simulink model "satellite3"  (R2025b)
settings: Solver=FixedStepAuto  StartTime=0.0  StopTime=100  FixedStep=dt  MinStep=0.0001  RelTol=1e-3
values from neighbouring files (symbols this model uses):
  A_mw = [ ... (first row only)    [init_params.m]
  A_w = [ ... (first row only)    [init_params.m]
  alpha1 = 0.1    [init_params.m]
  alpha2 = 0.1    [init_params.m]
  angle0 = eAR'    [init_params.m]
  area_d = 4    [init_params.m]
  area_m2 = 0.0127    [init_params.m]
  area_s = 2    [init_params.m]
  ARW_deg_per_sqrt_h = 0.01    [init_params.m]
  B_mw = [ ... (first row only)    [init_params.m]
  bat_bias_on = 0    [init_params.m]
  bat_bias_time = 0    [init_params.m]
  bat_bias_value = 0    [init_params.m]
  bat_cap_on = 0    [init_params.m]
  bat_cap_time = 0    [init_params.m]
  bat_cap_value = 1    [init_params.m]
  beta = 0.3    [init_params.m]
  beta1 = 0.01    [init_params.m]
  beta2 = 0.01    [init_params.m]
  bias0_deg_h = 0.01    [init_params.m]
  C_mw = [ ... (first row only)    [init_params.m]
  Cd = 2.2    [init_params.m]
  Cm = 0.01    [init_params.m]
  cmd_comm = 1    [init_params.m]
  comm_allow = 1    [init_params.m]
  cos_g_max = cos(gamma_max)    [init_params.m]
  Cr = 1.2    [init_params.m]
  cT_deg_on = 0    [init_params.m]
  cT_deg_time = 0    [init_params.m]
  cT_deg_value = 1    [init_params.m]
  cT_delay_on = 0    [init_params.m]
  cT_delay_time = 0    [init_params.m]
  cT_delay_value = 0    [init_params.m]
  cT_drop_on = 0    [init_params.m]
  cT_drop_time = 0    [init_params.m]
  cT_drop_value = 0    [init_params.m]
  cT_lock_on = 0    [init_params.m]
  cT_lock_time = 0    [init_params.m]
  d_c = 2e-5    (= 2e-05)    [init_params.m]
  d_f = 2e-5    (= 2e-05)    [init_params.m]
  D_max = 1    [init_params.m]
  D_thr = 0.4    [init_params.m]
  Delta_D = 0.001    [init_params.m]
  dP_th = 0.05    [init_params.m]
  dss_bias_on = 0    [init_params.m]
  dss_bias_time = 0    [init_params.m]
  dss_bias_value = [0;0;0]    [init_params.m]
  dss_delay_on = 0    [init_params.m]
  dss_delay_time = 0    [init_params.m]
  dss_delay_value = 0    [init_params.m]
  dss_drift_max = 0.1    [init_params.m]
  dss_drift_value = [0;0;0]    [init_params.m]
  dss_drop_on = 0    [init_params.m]
  dss_drop_time = 0    [init_params.m]
  dss_drop_value = [1;0;0]    [init_params.m]
  dss_lock_on = 0    [init_params.m]
  dss_lock_time = 0    [init_params.m]
  dt = 0.1    [init_params.m]
  earth_theta0 = 0    [init_params.m]
  epsilon = 0.01    [init_params.m]
  eT_deg_on = 0    [init_params.m]
  eT_deg_time = 0    [init_params.m]
  eT_deg_value = 1    [init_params.m]
  eT_delay_on = 0    [init_params.m]
  eT_delay_time = 0    [init_params.m]
  eT_delay_value = 0    [init_params.m]
  eT_drop_on = 0    [init_params.m]
  eT_drop_time = 0    [init_params.m]
  eT_drop_value = [0;0;0]    [init_params.m]
  eT_lock_on = 0    [init_params.m]
  eT_lock_time = 0    [init_params.m]
  eta = 0.7    [init_params.m]
  eta_buck = 0.9    [init_params.m]
  eta_et = 0.9    [init_params.m]
  eta_sspa = 0.35    [init_params.m]
  eta_twta = 0.35    [init_params.m]
  f = 2.2e9    (= 2200000000)    [init_params.m]
  f_n_hz = 400    [init_params.m]
  fov = 60*pi/180    (= 1.0471975512)    [init_params.m]
  g0 = 9.80665    [init_params.m]
  G0 = 1366.1    [init_params.m]
  G_sspa_dB = 20    [init_params.m]
  G_twta_dB = 20    [init_params.m]
  Gr_dB = 20    [init_params.m]
  Gt_dB = 3    [init_params.m]
  gyro_bias_on = 0    [init_params.m]
  gyro_bias_time = 0    [init_params.m]
  gyro_bias_value = [0;0;0]    [init_params.m]
  gyro_delay_on = 0    [init_params.m]
  gyro_delay_time = 0    [init_params.m]
  gyro_delay_value = 0    [init_params.m]
  gyro_drift_max = 0.1    [init_params.m]
  gyro_drift_value = [0;0;0]    [init_params.m]
  gyro_drop_on = 0    [init_params.m]
  gyro_drop_time = 0    [init_params.m]
  gyro_drop_value = [0;0;0]    [init_params.m]
  gyro_lock_on = 0    [init_params.m]
  gyro_lock_time = 0    [init_params.m]
  H = 50e3    (= 50000)    [init_params.m]
  h_max = Iw * rpm_max * sqrt(6)    [init_params.m]
  h_ref = 400e3    (= 400000)    [init_params.m]
  I_e = 11    [init_params.m]
  I_gate = 0.5    [init_params.m]
  I_triggle = 8    [init_params.m]
  i_w_max = 2    [init_params.m]
  i_w_min = -2    [init_params.m]
  initial_phase = 0    [init_params.m]
  Isp = 220    [init_params.m]
  Isp_et = 1500    [init_params.m]
  Iw = 0.02    [init_params.m]
  J2 = 1.08262668e-3    (= 0.00108262668)    [init_params.m]
  Jx = 10    [init_params.m]
  Jy = 12    [init_params.m]
  Jz = 8    [init_params.m]
  k_a = 4e-4    (= 0.0004)    [init_params.m]
  k_bias1_deg_h_per_C = 1    [init_params.m]
  k_bias2_deg_h_per_C = 0.0    (= 0)    [init_params.m]
  k_h = -0.05    [init_params.m]
  k_sf1_ppm = 1.0    (= 1)    [init_params.m]
  k_sf2_ppm = 0.0    (= 0)    [init_params.m]
  ... (+207 more)
libraries: matrix_library x25, simulink x14, nesl_utility x4, simulink_extras x3, fl_lib x3, ee_lib x1
(part 2 of 5)

== system satellite3/环境与动力学子系统/行星环境 ==
  x轴坐标 : Inport
  y轴坐标 : Inport  Port=2
  z轴坐标 : Inport  Port=3
  球心距 : Inport  Port=4
  ECI(vx) : Inport  Port=5
  ECI(vy) : Inport  Port=6
  ECI(vz) : Inport  Port=7
  日照标志 : Inport  Port=8
  星日单位向量 : Inport  Port=9
  Add : Sum  Inputs=+++
  Add1 : Sum  Inputs=+++
  Add2 : Sum  Inputs=+++
  J2摄动 : Subsystem
  大气阻力摄动 : Subsystem
  太阳光压摄动 : Subsystem
  ax : Outport
  ay : Outport  Port=2
  az : Outport  Port=3
  wires:
  x轴坐标/1 -> J2摄动/1(x轴坐标), 大气阻力摄动/1(x轴坐标)
  y轴坐标/1 -> J2摄动/2(y轴坐标), 大气阻力摄动/2(y轴坐标)
  z轴坐标/1 -> J2摄动/3(z轴坐标)
  球心距/1 -> 大气阻力摄动/3(球心距), J2摄动/4(球心距)
  ECI(vx)/1 -> 大气阻力摄动/4(vx)
  ECI(vy)/1 -> 大气阻力摄动/5(vy)
  ECI(vz)/1 -> 大气阻力摄动/6(vz)
  J2摄动/1(J2x) -> Add/1
  大气阻力摄动/1(Dx) -> Add/2
  Add/1 -> ax/1
  J2摄动/2(J2y) -> Add1/1
  大气阻力摄动/2(Dy) -> Add1/2
  Add1/1 -> ay/1
  J2摄动/3(J2z) -> Add2/1
  大气阻力摄动/3(Dz) -> Add2/2
  Add2/1 -> az/1
  太阳光压摄动/1(srp_x) -> Add/3
  太阳光压摄动/2(srp_y) -> Add1/3
  太阳光压摄动/3(srp_z) -> Add2/3
  星日单位向量/1 -> 太阳光压摄动/2(hat_r_ss)
  日照标志/1 -> 太阳光压摄动/1(sun_flag)

== system satellite3/电源子系统/充电调节器 ==
  负载电流 : Inport
  太阳能电池电流 : Inport  Port=2
  荷电状态 : Inport  Port=3
  1-SOC2 : Gain  Gain=0.2
  Add : Sum  Inputs=+-
  Add1 : Sum  Inputs=+-
  Constant : Constant  Value=0
  SOC1 : Constant  Value=SOC1
  SOC2 : Constant  Value=SOC2
  SOC_lt_SOC1 : RelationalOperator  Operator=>  OutDataTypeStr=boolean  RndMeth=Simplest  InputSameDT=off
  SOC_lt_SOC2 : RelationalOperator  Operator=>  OutDataTypeStr=boolean  RndMeth=Simplest  InputSameDT=off
  Scope1 : Scope
      settings: ActiveDisplayYMinimum=-0.1607142857142857  ActiveDisplayYMaximum=1.4464285714285716  DataLoggingVariableName=ScopeData43
  Switch : Switch  Criteria=u2 > Threshold  SaturateOnIntegerOverflow=off  InputSameDT=off
  Switch2 : Switch  Threshold=0.2  SaturateOnIntegerOverflow=off  InputSameDT=off
  涓流|稳流 : Switch  Criteria=u2 > Threshold  SaturateOnIntegerOverflow=off  InputSameDT=off
  涓流充电电流 : Constant  Value=0.3
  稳压充电电流 : Product
  稳流|稳压 : Switch  Criteria=u2 > Threshold  SaturateOnIntegerOverflow=off  InputSameDT=off
  稳流充电电流 : Constant  Value=0.6
  净充电电流 : Outport
  wires:
  [one] -> Add1/1
  SOC_lt_SOC2/1 -> 稳流|稳压/2
  1-SOC2/1 -> 稳流|稳压/3
  稳流充电电流/1 -> 稳流|稳压/1
  SOC_lt_SOC1/1 -> 涓流|稳流/2
  Add1/1 -> 1-SOC2/1
  SOC1/1 -> SOC_lt_SOC1/1
  SOC2/1 -> SOC_lt_SOC2/1
  涓流充电电流/1 -> 涓流|稳流/1
  稳流|稳压/1 -> 涓流|稳流/3
  涓流|稳流/1 -> 稳压充电电流/1
  Switch2/1 -> Scope1/1, Switch/3
  荷电状态/1 -> SOC_lt_SOC2/2, SOC_lt_SOC1/2, Switch2/2, Add1/2
  Constant/1 -> Switch2/3
  Add/1 -> Switch/2, 稳压充电电流/2, Switch2/1
  太阳能电池电流/1 -> Add/1
  负载电流/1 -> Add/2
  稳压充电电流/1 -> Switch/1
  Switch/1 -> 净充电电流/1

== system satellite3/电源子系统/太阳能板 ==
  note: V_bus 一旦跌到很低，I_load 变成极大，直接把系统拉飞
  note: 占比法计算负载电阻
      | $I_{load}=\frac{P_{cpl}}{V_{bus}}+\frac{V_{bus}}{R_{load}} \\ R_{load}=\frac{V_{bus,ref}^2}{P_R}=\frac{V_{bus,ref}^2}{\beta P_{load,max}}$
  note: 恒功率负载的“负阻抗”不稳定，当母线电压下降时，负载电流会增大，进一步拉低电压，容易引起母线电压振荡，因此添加电阻性负载
  note: 最简单的光生电流，后续可改为
      | $I_{pannel}=I_{ph}-I_0\left( e^{\frac{V_{pannel}+IR_s}{nV_t}} -1\right)-\frac{V_{pannel}+IR_s}{R_{sh}}$
  日照标志 : Inport
  q : Inport  Port=2
  星日单位矢量 : Inport  Port=3
  V_batt : Inport  Port=4
  电流差 : Inport  Port=5
  P_load : Inport  Port=6
  Gain2 : Gain  Gain=beta
  Gain3 : Gain  Gain=1/R_load
  Product3 : Product  Inputs=*/
  Relay : Relay  OnSwitchValue=V_uvlo_on  OffSwitchValue=V_uvlo_off
  Scope1 : Scope
      settings: ActiveDisplayYMinimum=26.370093999451154  ActiveDisplayYMaximum=30.950942722590582  DataLoggingVariableName=ScopeData29
  Scope3 : Scope
      settings: ActiveDisplayYMinimum=14  ActiveDisplayYMaximum=34  DataLoggingVariableName=ScopeData43
  Scope4 : Scope  NumInputPorts=3
      settings: ActiveDisplayYMinimum=-2.5150334771348364  ActiveDisplayYMaximum=7.0208781354201077  DataLoggingVariableName=ScopeData47
  Sum1 : Sum  Inputs=|++
  太阳板 : Subsystem
  数学保护 : Saturate  UpperLimit=50  LowerLimit=V_bus0
  母线故障 : Subsystem
  蓄电池充电电流 : Outport
  负载电流 : Outport  Port=2
  非欠压 : Outport  Port=3
  wires:
  太阳板/1(太阳板输出电流) -> 蓄电池充电电流/1, Scope4/1
  Sum1/1 -> Scope4/3, 负载电流/1  "I_load"
  q/1 -> 太阳板/1(q)
  日照标志/1 -> 太阳板/2(日照标志)
  母线故障/1(故障值) -> Scope1/1, Relay/1, 太阳板/4(母线电压), 数学保护/1, Gain3/1  "V_bus"
  星日单位矢量/1 -> 太阳板/3(星日单位矢量)
  Gain2/1 -> Product3/1
  Product3/1 -> Sum1/1
  Gain3/1 -> Sum1/2
  数学保护/1 -> Product3/2
  Relay/1 -> 非欠压/1
  P_load/1 -> Gain2/1
  电流差/1 -> Scope4/2
  V_batt/1 -> 母线故障/1(原值)

== system satellite3/电源子系统/姿态确认与控制功耗 ==
  SOC : Inport
  adcs_load : Inport  Port=2
  not_shed : Inport  Port=3
  0.01 : Constant  Commented=on  Value=0.01
  1 : Constant
  AND1 : Logic  Inputs=5  AllPortsSameDT=off  OutDataTypeStr=boolean
  AND2 : Logic  AllPortsSameDT=off  OutDataTypeStr=boolean
  Add2 : Sum
  SOC_adcs_1/0 : Relay  OnSwitchValue=SOC_low_adcs + 0.02  OffSwitchValue=SOC_low_adcs  OutDataTypeStr=boolean
  Switch : Switch  Criteria=u2 > Threshold  Threshold=0.5  SaturateOnIntegerOverflow=off  InputSameDT=off
  T_gt_001 : RelationalOperator  Commented=on  Operator=<=  OutDataTypeStr=boolean  RndMeth=Simplest  InputSameDT=off
  姿态开时负载功耗 : Constant  Value=P_adcs
  adcs_on : Outport
  P_adcs : Outport  Port=2
  wires:
  Switch/1 -> P_adcs/1
  adcs_load/1 -> Add2/1, T_gt_001/2
  AND2/1 -> Switch/2, adcs_on/1
  Add2/1 -> Switch/1
  0.01/1 -> T_gt_001/1
  姿态开时负载功耗/1 -> Add2/2
  [zero] -> Switch/3
  SOC/1 -> SOC_adcs_1/0/1
  SOC_adcs_1/0/1 -> AND2/2
  1/1 -> AND2/1

== system satellite3/电源子系统/推进子系统功耗 ==
  SOC : Inport
  prop_load : Inport  Port=2
  not_shed : Inport  Port=3
  2 : Constant
  AND : Logic  AllPortsSameDT=off  OutDataTypeStr=boolean
  SOC_prop_1/0 : Relay  OnSwitchValue=SOC_low_prop + 0.02  OffSwitchValue=SOC_low_prop  OutDataTypeStr=boolean
  Switch : Switch  Criteria=u2 > Threshold  Threshold=0.5  SaturateOnIntegerOverflow=off  InputSameDT=off
  P_prop : Outport
  prop_on : Outport  Port=2
  wires:
  SOC/1 -> SOC_prop_1/0/1
  AND/1 -> prop_on/1, Switch/2
  Switch/1 -> P_prop/1
  prop_load/1 -> Switch/1
  [zero] -> Switch/3
  SOC_prop_1/0/1 -> AND/1
  2/1 -> AND/2

== system satellite3/电源子系统/蓄电池组 ==
  净充电电流 : Inport
  Add3 : Sum
  Ah2As : Gain  Gain=1/3600
  Constant : Constant  Value=Qbat
  D : Gain  Gain=Rb
  Fcn : Fcn  Expr=24+9*u
  Fcn1 : Fcn  Expr=-7.5*u^3+15*u^2+3.5*u+24
  I_delay : Memory  LinearizeAsDelay=on
  Product : Product  Inputs=*/
  Scope1 : Scope
      settings: ActiveDisplayYMinimum=29.158033567408072  ActiveDisplayYMaximum=29.963419336128545  DataLoggingVariableName=ScopeData27
  Scope2 : Scope
      settings: ActiveDisplayYMinimum=0.59993300420194839  ActiveDisplayYMaximum=0.60060296218246534  DataLoggingVariableName=ScopeData9
  Scope3 : Scope
      settings: ActiveDisplayYMinimum=-2.9294047342041475E-5  ActiveDisplayYMaximum=4.7292744475508951E-5  DataLoggingVariableName=ScopeData51
  int_Q : Integrator  InitialCondition=SOC0*Qbat  LimitOutput=on  UpperSaturationLimit=Qbat  LowerSaturationLimit=0
  蓄电池组故障 : Subsystem
  V_batt : Outport
  电流差 : Outport  Port=2
  SOC : Outport  Port=3
  wires:
  Add3/1 -> V_batt/1
  净充电电流/1 -> I_delay/1
  Fcn1/1 -> Scope1/1, Add3/2
  Product/1 -> Fcn1/1, Scope2/1, SOC/1
  D/1 -> Add3/1
  I_delay/1 -> 电流差/1, Ah2As/1, D/1
  int_Q/1 -> Product/1, Scope3/1
  Ah2As/1 -> int_Q/1
  Constant/1 -> 蓄电池组故障/1(原值)
  蓄电池组故障/1(故障值) -> Product/2

== system satellite3/电源子系统/通信子系统功耗 ==
  note: 因为阴影期 电源更紧张 ：太阳板发电为 0，所有功耗都由电池承担。通信通常是大功耗载荷之一（例如几十瓦到上百瓦），如果阴影期仍高占空比通信，SOC 会更快下滑，导致系统触发保护（关载荷/进 Safe Mode）
  SOC : Inport
  Vizlit : Inport  Port=2
  sunlit : Inport  Port=3
  not_shed : Inport  Port=4
  cmd_comm_on : Inport  Port=5
  1 : Constant
  3 : Constant
  4 : Constant
  AND1 : Logic  Inputs=5  AllPortsSameDT=off  OutDataTypeStr=boolean
  SOC_comm_1/0 : Relay  OnSwitchValue=SOC_low_comm + 0.02  OffSwitchValue=SOC_low_comm
  Switch : Switch  Criteria=u2 > Threshold  Threshold=0.5  SaturateOnIntegerOverflow=off  InputSameDT=off
  通信开时负载功耗 : Constant  Value=P_comm
  comm_on : Outport
  通信功耗 : Outport  Port=2
  wires:
  AND1/1 -> Switch/2, comm_on/1
  sunlit/1 -> AND1/3
  通信开时负载功耗/1 -> Switch/1
  SOC_comm_1/0/1 -> AND1/1
  Switch/1 -> 通信功耗/1
  SOC/1 -> SOC_comm_1/0/1
  Vizlit/1 -> AND1/2
  [zero] -> Switch/3
  cmd_comm_on/1 -> AND1/5
  1/1 -> AND1/4

== system satellite3/通信子系统/SSPA ==
  tx_on : Inport
  Gain : Gain  Gain=0.1
  Gain1 : Gain  Gain=1/eta_sspa
  Math Function : Math  Operator=10^u
  Saturation : Saturate  UpperLimit=P_sspa_dBW  LowerLimit=0
  Sum : Sum  Inputs=|++
  Switch : Switch  Criteria=u2 > Threshold  SaturateOnIntegerOverflow=off  InputSameDT=off
  dbW : Constant  Value=-100
  前级驱动功率 : Constant  Value=P_in_driver_dBW
  小信号增益 : Constant  Value=G_sspa_dB
  Pt_dBW : Outport
  load : Outport  Port=2
  wires:
  前级驱动功率/1 -> Sum/1
  小信号增益/1 -> Sum/2
  Sum/1 -> Saturation/1
  Saturation/1 -> Switch/1
  tx_on/1 -> Switch/2
  dbW/1 -> Switch/3
  Math Function/1 -> Gain1/1
  Gain/1 -> Math Function/1
  Switch/1 -> Gain/1, Pt_dBW/1
  Gain1/1 -> load/1

== system satellite3/通信子系统/TWTA ==
  note: TWTA 往往不是瞬时可用。比如：
      | 发射指令来了后开始计时
      | 计时大于 5 s 才允许输出功率
      | 这会比 SSPA 更贴近工程。
  tx_on : Inport
  Delay1 : Delay  DelayLength=5/dt
  Gain : Gain  Gain=0.1
  Gain1 : Gain  Gain=1/eta_twta
  Math Function : Math  Operator=10^u
  Saturation : Saturate  UpperLimit=P_twta_dBW  LowerLimit=0
  Sum : Sum  Inputs=|++
  Switch : Switch  Criteria=u2 > Threshold  SaturateOnIntegerOverflow=off  InputSameDT=off
  dbW : Constant  Value=-100
  前级驱动功率 : Constant  Value=P_in_driver_dBW
  小信号增益 : Constant  Value=G_twta_dB
  Pt_dBW : Outport
  load : Outport  Port=2
  wires:
  dbW/1 -> Switch/3
  Saturation/1 -> Switch/1
  Sum/1 -> Saturation/1
  小信号增益/1 -> Sum/2
  前级驱动功率/1 -> Sum/1
  Gain1/1 -> load/1
  Math Function/1 -> Gain1/1
  Gain/1 -> Math Function/1
  Delay1/1 -> Pt_dBW/1, Gain/1
  tx_on/1 -> Switch/2
  Switch/1 -> Delay1/1

== system satellite3/通信子系统/向量模长-r ==
  u1 : Inport
  u2 : Inport  Port=2
  u3 : Inport  Port=3
  Add : Sum  Inputs=+++
  Sqrt : Sqrt
  Square : Math  Operator=square
  Square1 : Math  Operator=square
  Square2 : Math  Operator=square
  |u| : Outport
  wires:
  u1/1 -> Square/1
  u2/1 -> Square1/1
  u3/1 -> Square2/1
  Square/1 -> Add/1
  Square1/1 -> Add/2
  Square2/1 -> Add/3
  Add/1 -> Sqrt/1
  Sqrt/1 -> |u|/1

== system satellite3/姿态确定与控制系统/三轴PD控制器/共轭 ==
  u : Inport
  -q1 : Gain  Gain=-1
  -q2 : Gain  Gain=-1
  -q3 : Gain  Gain=-1
  Demux : Demux
  Mux : Mux
  u^-1 : Outport
  wires:
  Mux/1 -> u^-1/1
  Demux/1 -> Mux/1
  Demux/2 -> -q1/1
  -q1/1 -> Mux/2
  Demux/3 -> -q2/1
  -q2/1 -> Mux/3
  Demux/4 -> -q3/1
  -q3/1 -> Mux/4
  u/1 -> Demux/1

== system satellite3/姿态确定与控制系统/三轴PD控制器/四元数乘法 ==
  Q1 : Inport
  Q2 : Inport  Port=2
  Add : Sum  Inputs=3
  Cross Product : matrix_library/Cross Product
  Demux : Demux
  Demux1 : Demux
  Dot Product : DotProduct  OutDataTypeStr=Inherit: Inherit via internal rule
  Mux : Mux  Inputs=2
  Mux1 : Mux  Inputs=3
  Mux2 : Mux  Inputs=3
  Product : Product
  Product1 : Product
  Product2 : Product
  Sum : Sum  Inputs=|+-
  四元数旋转偏差 : Outport
  wires:
  Q1/1 -> Demux/1
  Q2/1 -> Demux1/1
  Mux/1 -> 四元数旋转偏差/1
  Product/1 -> Sum/1
  Demux/1 -> Product1/1, Product/1
  Mux1/1 -> Dot Product/1, Cross Product/1, Product2/2
  Demux1/1 -> Product2/1, Product/2
  Mux2/1 -> Cross Product/2, Dot Product/2, Product1/2
  Sum/1 -> Mux/1
  Dot Product/1 -> Sum/2
  Product2/1 -> Add/2
  Product1/1 -> Add/1
  Cross Product/1 -> Add/3
  Add/1 -> Mux/2
  Demux/2 -> Mux1/1
  Demux/3 -> Mux1/2
  Demux/4 -> Mux1/3
  Demux1/2 -> Mux2/1
  Demux1/3 -> Mux2/2
  Demux1/4 -> Mux2/3

== system satellite3/姿态确定与控制系统/三轴PD控制器/四元数归一化 ==
  In1 : Inport
  Demux1 : Demux
  Mux1 : Mux
  Product{2..5} (4 alike) : Product  Inputs=*/
  向量模长-q : Subsystem
  Out1 : Outport
  wires:
  Demux1/4 -> Product5/1, 向量模长-q/4(u3)
  Product5/1 -> Mux1/4  "q3"
  Demux1/2 -> 向量模长-q/2(u1), Product3/1
  向量模长-q/1(|u|) -> Product3/2, Product4/2, Product5/2, Product2/2
  Demux1/1 -> 向量模长-q/1(u0), Product2/1
  Demux1/3 -> 向量模长-q/3(u2), Product4/1
  Product3/1 -> Mux1/2  "q1"
  Product2/1 -> Mux1/1  "q0"
  Product4/1 -> Mux1/3  "q2"
  Mux1/1 -> Out1/1
  In1/1 -> Demux1/1

== system satellite3/姿态确定与控制系统/三轴姿态动力学子系统/rlg_p ==
  p : Inport
  Lamb激光动力学 : Subsystem
  Sum : Sum  Inputs=+-|
  Terminator : Terminator
  几何参数 : Subsystem
  噪声模型 : Subsystem
  控模与扫模逻辑 : Subsystem
  机械抖动 : Subsystem  Commented=on
  热模型 : Subsystem
  环境温度 : Sin  Amplitude=10  Bias=25  Frequency=(2*pi)/3600  SampleTime=0
  hat_p : Outport
  wires:
  控模与扫模逻辑/1(扫模电压) -> Lamb激光动力学/5(扫模电压)
  Lamb激光动力学/1(相位差变化率) -> 噪声模型/2(相位差变化率)
  热模型/2(温度标度因数) -> Lamb激光动力学/2(温度标度因数)
  噪声模型/1(测量角速度) -> Sum/2, hat_p/1  "测量角速度"
  几何参数/1(标度因数) -> 噪声模型/1(标度因数), 热模型/2(几何标度因数)
  p/1 -> Lamb激光动力学/1(本体角速度), Sum/1  "本体角速度"
  机械抖动/1(抖动角速度) -> Lamb激光动力学/4(抖动角速度)
  热模型/3(温度零偏) -> Lamb激光动力学/3(零偏速率)
  环境温度/1 -> 热模型/1(环境温度-°C)
  Lamb激光动力学/2(光强) -> 控模与扫模逻辑/1(光强)
  Sum/1 -> Terminator/1

== system satellite3/姿态确定与控制系统/三轴姿态动力学子系统/rlg_q ==
  q : Inport
  Lamb激光动力学 : Subsystem
  Sum : Sum  Inputs=+-|
  Terminator : Terminator
  几何参数 : Subsystem
  噪声模型 : Subsystem
  控模与扫模逻辑 : Subsystem
  机械抖动 : Subsystem  Commented=on
  热模型 : Subsystem
  环境温度 : Sin  Amplitude=10  Bias=25  Frequency=(2*pi)/3600  SampleTime=0
  hat_q : Outport
  wires:
  Sum/1 -> Terminator/1
  Lamb激光动力学/2(光强) -> 控模与扫模逻辑/1(光强)
  环境温度/1 -> 热模型/1(环境温度-°C)
  热模型/3(温度零偏) -> Lamb激光动力学/3(零偏速率)
  机械抖动/1(抖动角速度) -> Lamb激光动力学/4(抖动角速度)
  q/1 -> Sum/1, Lamb激光动力学/1(本体角速度)  "本体角速度"
  几何参数/1(标度因数) -> 热模型/2(几何标度因数), 噪声模型/1(标度因数)
  噪声模型/1(测量角速度) -> hat_q/1, Sum/2  "测量角速度"
  热模型/2(温度标度因数) -> Lamb激光动力学/2(温度标度因数)
  Lamb激光动力学/1(相位差变化率) -> 噪声模型/2(相位差变化率)
  控模与扫模逻辑/1(扫模电压) -> Lamb激光动力学/5(扫模电压)

== system satellite3/姿态确定与控制系统/三轴姿态动力学子系统/rlg_r ==
  r : Inport
  Lamb激光动力学 : Subsystem
  Sum : Sum  Inputs=+-|
  Terminator : Terminator
  几何参数 : Subsystem
  噪声模型 : Subsystem
  控模与扫模逻辑 : Subsystem
  机械抖动 : Subsystem  Commented=on
  热模型 : Subsystem
  环境温度 : Sin  Amplitude=10  Bias=25  Frequency=(2*pi)/3600  SampleTime=0
  hat_r : Outport
  wires:
  控模与扫模逻辑/1(扫模电压) -> Lamb激光动力学/5(扫模电压)
  Lamb激光动力学/1(相位差变化率) -> 噪声模型/2(相位差变化率)
  热模型/2(温度标度因数) -> Lamb激光动力学/2(温度标度因数)
  噪声模型/1(测量角速度) -> Sum/2, hat_r/1  "测量角速度"
  几何参数/1(标度因数) -> 噪声模型/1(标度因数), 热模型/2(几何标度因数)
  r/1 -> Lamb激光动力学/1(本体角速度), Sum/1  "本体角速度"
  机械抖动/1(抖动角速度) -> Lamb激光动力学/4(抖动角速度)
  热模型/3(温度零偏) -> Lamb激光动力学/3(零偏速率)
  环境温度/1 -> 热模型/1(环境温度-°C)
  Lamb激光动力学/2(光强) -> 控模与扫模逻辑/1(光强)
  Sum/1 -> Terminator/1

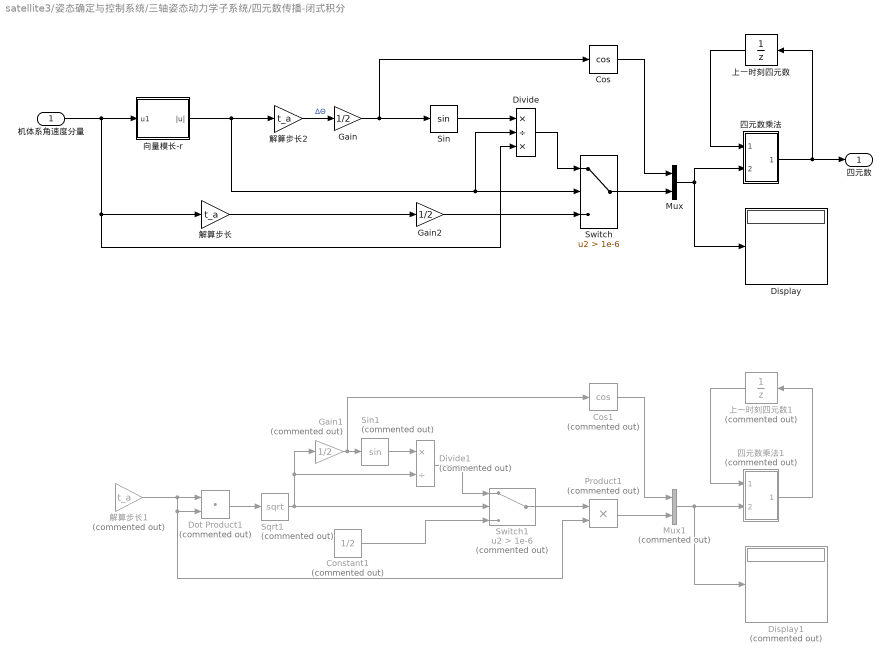
== system satellite3/姿态确定与控制系统/三轴姿态动力学子系统/四元数传播-闭式积分 ==
  机体系角速度分量 : Inport
  Constant1 : Constant  Commented=on  Value=1/2
  Cos : Trigonometry  Operator=cos
  Cos1 : Trigonometry  Commented=on  Operator=cos
  Display : Display
  Display1 : Display  Commented=on
  Divide : Product  Inputs=*/*
  Divide1 : Product  Commented=on  Inputs=*/
  Dot Product1 : DotProduct  Commented=on  OutDataTypeStr=Inherit: Inherit via internal rule
  Gain : Gain  Gain=1/2
  Gain1 : Gain  Commented=on  Gain=1/2
  Gain2 : Gain  Gain=1/2
  Mux : Mux  Inputs=2
  Mux1 : Mux  Commented=on  Inputs=2
  Product1 : Product  Commented=on
  Sin : Trigonometry
  Sin1 : Trigonometry  Commented=on
  Sqrt1 : Sqrt  Commented=on
  Switch : Switch  Criteria=u2 > Threshold  Threshold=1e-6  SaturateOnIntegerOverflow=off  InputSameDT=off
  Switch1 : Switch  Commented=on  Criteria=u2 > Threshold  Threshold=1e-6  SaturateOnIntegerOverflow=off  InputSameDT=off
  上一时刻四元数 : UnitDelay  InitialCondition=Q0  SampleTime=t_a  HasFrameUpgradeWarning=on
  上一时刻四元数1 : UnitDelay  Commented=on  InitialCondition=Q0  SampleTime=t_a  HasFrameUpgradeWarning=on
  向量模长-r : Subsystem
  四元数乘法 : Subsystem
  四元数乘法1 : Subsystem  Commented=on
  解算步长 : Gain  Gain=t_a
  解算步长1 : Gain  Commented=on  Gain=t_a
  解算步长2 : Gain  Gain=t_a
  四元数 : Outport
  wires:
  机体系角速度分量/1 -> 向量模长-r/1(u1), Divide/3, 解算步长/1
  解算步长/1 -> Gain2/1
  Gain/1 -> Sin/1, Cos/1
  Cos/1 -> Mux/1
  Mux/1 -> 四元数乘法/2(Q2), Display/1
  四元数乘法/1(Q*) -> 四元数/1, 上一时刻四元数/1
  上一时刻四元数/1 -> 四元数乘法/1(Q1)
  Mux1/1 -> Display1/1, 四元数乘法1/2(Q2)
  Sqrt1/1 -> Gain1/1, Divide1/2, Switch1/2
  解算步长1/1 -> Dot Product1/1, Product1/2, Dot Product1/2
  四元数乘法1/1(Q*) -> 上一时刻四元数1/1
  Switch1/1 -> Product1/1
  Gain1/1 -> Cos1/1, Sin1/1
  Constant1/1 -> Switch1/3
  Sin1/1 -> Divide1/1
  上一时刻四元数1/1 -> 四元数乘法1/1(Q1)
  Divide1/1 -> Switch1/1
  Dot Product1/1 -> Sqrt1/1
  Cos1/1 -> Mux1/1
  Product1/1 -> Mux1/2
  Sin/1 -> Divide/1
  Gain2/1 -> Switch/3
  向量模长-r/1(|u|) -> 解算步长2/1, Switch/2, Divide/2
  解算步长2/1 -> Gain/1  "ΔΘ"
  Switch/1 -> Mux/2
  Divide/1 -> Switch/1

== system satellite3/姿态确定与控制系统/三轴姿态动力学子系统/姿态解算 ==
  陀螺测量角速度 : Inport
  w_true : Inport  Port=2
  hat_ss_i : Inport  Port=3
  hat_r_o : Inport  Port=4
  Scope3 : Scope
      settings: ActiveDisplayYMinimum=-1.0125551437729807  ActiveDisplayYMaximum=2.1731621670894694  DataLoggingVariableName=ScopeData35
  Scope4 : Scope
      settings: ActiveDisplayYMinimum=-0.47759610261772045  ActiveDisplayYMaximum=2.1137222736277739  DataLoggingVariableName=ScopeData36
  Sum : Sum  Inputs=|+-
  四元数传播-欧拉法 : Subsystem
  星敏 : Subsystem
  欧拉数传播 : Subsystem
  欧拉角 : MATLAB Function  TreatAsAtomicUnit=on
  简化互补滤波器 : Subsystem
  解算角速度 : Outport
  三轴欧拉角 : Outport  Port=2
  解算四元数 : Outport  Port=3
  q_true : Outport  Port=4
  wires:
  w_true/1 -> 四元数传播-欧拉法/1(机体系角速度分量), 欧拉数传播/1(机体系角速度分量)
  四元数传播-欧拉法/1(四元数) -> 星敏/1(q_true), 简化互补滤波器/6(q_true), 欧拉角/1(Q), q_true/1
  Sum/1 -> 解算角速度/1
  星敏/2(st_valid) -> 简化互补滤波器/3(星敏有效标志)
  陀螺测量角速度/1 -> Sum/1, 简化互补滤波器/1(陀螺测量角速度)
  欧拉数传播/1(三轴欧拉角) -> Scope3/1
  欧拉角/1(angle) -> 三轴欧拉角/1, Scope4/1
  hat_ss_i/1 -> 简化互补滤波器/4(hat_ss_i)
  hat_r_o/1 -> 简化互补滤波器/5(hat_r_o)
  简化互补滤波器/1(陀螺偏置估计) -> Sum/2
  简化互补滤波器/2(预测姿态) -> 解算四元数/1
  星敏/1(q_star) -> 简化互补滤波器/2(星敏测量姿态)

== system satellite3/姿态确定与控制系统/三轴姿态动力学子系统/陀螺仪故障 ==
  原值 : Inport
  Add : Sum  Inputs=+++++
  Sum : Sum  Inputs=|++
  偏差故障 : Subsystem
  延迟故障 : Subsystem
  掉线故障 : Subsystem
  漂移故障 : Subsystem
  锁死故障 : Subsystem
  故障值 : Outport
  wires:
  原值/1 -> 延迟故障/1(原值), 掉线故障/1(原值), 锁死故障/1(原值), Sum/1
  Sum/1 -> 故障值/1
  Add/1 -> Sum/2
  偏差故障/1(故障值注入) -> Add/1
  漂移故障/1(故障值注入) -> Add/2
  锁死故障/1(故障值注入) -> Add/3
  掉线故障/1(故障值注入) -> Add/4
  延迟故障/1(故障值注入) -> Add/5

== system satellite3/姿态确定与控制系统/金字塔反作用轮组件/反作用轮组件 ==
  note: 摩擦模型添加，但未接入
  指令力矩 : Inport
  Bus Creator : BusCreator  Inputs=4  OutDataTypeStr=Bus: wheel
  Demux : Demux
  反作用轮1 : Subsystem
  反作用轮2 : Subsystem
  反作用轮3 : Subsystem
  反作用轮4 : Subsystem
  Wheel : Outport
  wires:
  指令力矩/1 -> Demux/1
  Bus Creator/1 -> Wheel/1
  Demux/1 -> 反作用轮1/1(指令力矩)
  Demux/2 -> 反作用轮2/1(指令力矩)
  Demux/3 -> 反作用轮3/1(指令力矩)
  Demux/4 -> 反作用轮4/1(指令力矩)
  反作用轮1/1(Wheel) -> Bus Creator/1  "wheel1"
  反作用轮2/1(Wheel) -> Bus Creator/2  "wheel2"
  反作用轮3/1(Wheel) -> Bus Creator/3  "wheel3"
  反作用轮4/1(Wheel) -> Bus Creator/4  "wheel4"

== system satellite3/姿态确定与控制系统/金字塔反作用轮组件/饱和标志 ==
  H : Inport
  Abs1 : Abs  SaturateOnIntegerOverflow=off
  Abs2 : Abs  SaturateOnIntegerOverflow=off
  Abs3 : Abs  SaturateOnIntegerOverflow=off
  Constant : Constant  Value=[0;0;0]
  Demux : Demux  Outputs=3
  Gain : Gain  Gain=k_h
  Mux : Mux  Inputs=3
  Relay : Relay  OnSwitchValue=h_max  OffSwitchValue=h_max *sf_factor
  Relay1 : Relay  OnSwitchValue=h_max  OffSwitchValue=h_max * sf_factor
  Relay2 : Relay  OnSwitchValue=h_max  OffSwitchValue=h_max * sf_factor
  Switch : Switch  Criteria=u2 > Threshold  Threshold=0.5  SaturateOnIntegerOverflow=off  InputSameDT=off
  Switch1 : Switch  Criteria=u2 > Threshold  Threshold=0.5  SaturateOnIntegerOverflow=off  InputSameDT=off
  Switch2 : Switch  Criteria=u2 > Threshold  Threshold=0.5  SaturateOnIntegerOverflow=off  InputSameDT=off
  指令退饱和力矩 : Outport
  wires:
  Demux/1 -> Switch/1, Abs1/1
  Abs1/1 -> Relay/1
  H/1 -> Demux/1
  Abs2/1 -> Relay1/1
  Demux/2 -> Switch1/1, Abs2/1
  Demux/3 -> Switch2/1, Abs3/1
  Abs3/1 -> Relay2/1
  Relay/1 -> Switch/2
  [zero] -> Switch2/3, Switch1/3, Switch/3
  Relay1/1 -> Switch1/2
  Relay2/1 -> Switch2/2
  Switch/1 -> Mux/1
  Switch1/1 -> Mux/2
  Switch2/1 -> Mux/3
  Gain/1 -> 指令退饱和力矩/1
  Constant/1 -> Gain/1

== system satellite3/推进子系统/化推/推力故障 ==
  原值 : Inport
  Add : Sum  Inputs=4
  Sum : Sum  Inputs=|++
  延迟故障 : Subsystem
  掉线故障 : Subsystem
  退化故障 : Subsystem
  锁死故障 : Subsystem
  故障值 : Outport
  wires:
  退化故障/1(故障值注入) -> Add/1
  Add/1 -> Sum/2
  Sum/1 -> 故障值/1
  原值/1 -> Sum/1, 延迟故障/1(原值), 锁死故障/1(原值), 掉线故障/1(原值), 退化故障/1(原值)
  掉线故障/1(故障值注入) -> Add/2
  锁死故障/1(故障值注入) -> Add/3
  延迟故障/1(故障值注入) -> Add/4

== system satellite3/推进子系统/电推/向量模长-P ==
  u : Inport
  Add : Sum  Inputs=+++
  Demux : Demux  Outputs=3
  Sqrt : Sqrt
  Square : Math  Operator=square
  Square1 : Math  Operator=square
  Square2 : Math  Operator=square
  |u| : Outport
  wires:
  u/1 -> Demux/1
  Demux/1 -> Square/1
  Sqrt/1 -> |u|/1
  Add/1 -> Sqrt/1
  Square2/1 -> Add/3
  Square1/1 -> Add/2
  Square/1 -> Add/1
  Demux/3 -> Square2/1
  Demux/2 -> Square1/1

== system satellite3/推进子系统/电推/向量模长-T ==
  u : Inport
  Add : Sum  Inputs=+++
  Demux : Demux  Outputs=3
  Sqrt : Sqrt
  Square : Math  Operator=square
  Square1 : Math  Operator=square
  Square2 : Math  Operator=square
  |u| : Outport
  wires:
  Demux/2 -> Square1/1
  Demux/3 -> Square2/1
  Square/1 -> Add/1
  Square1/1 -> Add/2
  Square2/1 -> Add/3
  Add/1 -> Sqrt/1
  Sqrt/1 -> |u|/1
  Demux/1 -> Square/1
  u/1 -> Demux/1

== system satellite3/推进子系统/电推/推力故障 ==
  原值 : Inport
  Add : Sum  Inputs=4
  Sum : Sum  Inputs=|++
  延迟故障 : Subsystem
  掉线故障 : Subsystem
  退化故障 : Subsystem
  锁死故障 : Subsystem
  故障值 : Outport
  wires:
  退化故障/1(故障值注入) -> Add/1
  Add/1 -> Sum/2
  Sum/1 -> 故障值/1
  原值/1 -> Sum/1, 延迟故障/1(原值), 锁死故障/1(原值), 掉线故障/1(原值), 退化故障/1(原值)
  掉线故障/1(故障值注入) -> Add/2
  锁死故障/1(故障值注入) -> Add/3
  延迟故障/1(故障值注入) -> Add/4

== system satellite3/推进子系统/电推/电推惯性 ==
  指令 : Inport
  Demux : Demux  Outputs=3
  Mux : Mux  Inputs=3
  Transfer Fcn : TransferFcn  Denominator=[tau_et 1]
  Transfer Fcn1 : TransferFcn  Denominator=[tau_et 1]
  Transfer Fcn2 : TransferFcn  Denominator=[tau_et 1]
  实际 : Outport
  wires:
  指令/1 -> Demux/1
  Demux/1 -> Transfer Fcn/1
  Demux/2 -> Transfer Fcn1/1
  Demux/3 -> Transfer Fcn2/1
  Transfer Fcn/1 -> Mux/1
  Transfer Fcn1/1 -> Mux/2
  Transfer Fcn2/1 -> Mux/3
  Mux/1 -> 实际/1

== system satellite3/测控子系统/视线角标志/余弦夹角 ==
  u1 : Inport
  u2 : Inport  Port=2
  Demux : Demux  Outputs=3
  Demux1 : Demux  Outputs=3
  Dot Product : DotProduct  OutDataTypeStr=Inherit: Inherit via internal rule
  余弦夹角 : Product  Inputs=/*/
  向量模长-r1 : Subsystem
  向量模长-r2 : Subsystem
  cos(γ) : Outport
  wires:
  向量模长-r2/1(|u|) -> 余弦夹角/3
  Demux/3 -> 向量模长-r1/3(u3)
  Demux/2 -> 向量模长-r1/2(u2)
  Dot Product/1 -> 余弦夹角/2
  Demux/1 -> 向量模长-r1/1(u1)
  向量模长-r1/1(|u|) -> 余弦夹角/1
  u2/1 -> Dot Product/2, Demux1/1
  Demux1/1 -> 向量模长-r2/1(u1)
  Demux1/2 -> 向量模长-r2/2(u2)
  Demux1/3 -> 向量模长-r2/3(u3)
  u1/1 -> Dot Product/1, Demux/1
  余弦夹角/1 -> cos(γ)/1

== system satellite3/环境与动力学子系统/J2000模型/向量模长-r_ss ==
  u : Inport
  Add : Sum  Inputs=3
  Demux : Demux  Outputs=3
  Sqrt : Sqrt
  Square : Math  Operator=square
  Square1 : Math  Operator=square
  Square2 : Math  Operator=square
  |u| : Outport
  wires:
  u/1 -> Demux/1
  Demux/2 -> Square1/1
  Demux/3 -> Square2/1
  Square/1 -> Add/1
  Square1/1 -> Add/2
  Square2/1 -> Add/3
  Add/1 -> Sqrt/1
  Sqrt/1 -> |u|/1
  Demux/1 -> Square/1

== system satellite3/环境与动力学子系统/OrbitElements/向量模长-e ==
  u1 : Inport
  u2 : Inport  Port=2
  u3 : Inport  Port=3
  Add : Sum  Inputs=+++
  Sqrt : Sqrt
  Square : Math  Operator=square
  Square1 : Math  Operator=square
  Square2 : Math  Operator=square
  |u| : Outport
  wires:
  u1/1 -> Square/1
  u2/1 -> Square1/1
  u3/1 -> Square2/1
  Square/1 -> Add/1
  Square1/1 -> Add/2
  Square2/1 -> Add/3
  Add/1 -> Sqrt/1
  Sqrt/1 -> |u|/1

== system satellite3/环境与动力学子系统/OrbitElements/向量模长-h ==
  u1 : Inport
  u2 : Inport  Port=2
  u3 : Inport  Port=3
  Add : Sum  Inputs=+++
  Sqrt : Sqrt
  Square : Math  Operator=square
  Square1 : Math  Operator=square
  Square2 : Math  Operator=square
  |u| : Outport
  wires:
  Sqrt/1 -> |u|/1
  Add/1 -> Sqrt/1
  Square2/1 -> Add/3
  Square1/1 -> Add/2
  Square/1 -> Add/1
  u3/1 -> Square2/1
  u2/1 -> Square1/1
  u1/1 -> Square/1

== system satellite3/环境与动力学子系统/OrbitElements/向量模长-r ==
  u1 : Inport
  u2 : Inport  Port=2
  u3 : Inport  Port=3
  Add : Sum  Inputs=+++
  Sqrt : Sqrt
  Square : Math  Operator=square
  Square1 : Math  Operator=square
  Square2 : Math  Operator=square
  |u| : Outport
  wires:
  u1/1 -> Square/1
  u2/1 -> Square1/1
  u3/1 -> Square2/1
  Square/1 -> Add/1
  Square1/1 -> Add/2
  Square2/1 -> Add/3
  Add/1 -> Sqrt/1
  Sqrt/1 -> |u|/1

== system satellite3/环境与动力学子系统/OrbitElements/向量模长-v ==
  u1 : Inport
  u2 : Inport  Port=2
  u3 : Inport  Port=3
  Add : Sum  Inputs=+++
  Sqrt : Sqrt
  Square : Math  Operator=square
  Square1 : Math  Operator=square
  Square2 : Math  Operator=square
  |u| : Outport
  wires:
  Sqrt/1 -> |u|/1
  Add/1 -> Sqrt/1
  Square2/1 -> Add/3
  Square1/1 -> Add/2
  Square/1 -> Add/1
  u3/1 -> Square2/1
  u2/1 -> Square1/1
  u1/1 -> Square/1

== system satellite3/环境与动力学子系统/行星环境/J2摄动 ==
  note: $a_{J2}=\frac{3}{2}J_2\mu\frac{R_e^2}{r^5} \left[\begin{array}{ccc} x(5\frac{z^2}{r^2}-1)\\ y(5\frac{z^2}{r^2}-1)\\ z(5\frac{z^2}{r^2}-3) \end{array}\right]$
  x轴坐标 : Inport
  y轴坐标 : Inport  Port=2
  z轴坐标 : Inport  Port=3
  球心距 : Inport  Port=4
  J2 : Constant  Value=J2
  J2_x : Product  Inputs=3
  J2_y : Product  Inputs=3
  J2_z : Product  Inputs=3
  Product : Product  Inputs=/****
  Re : Constant  Value=Re
  Re2 : Math  Operator=square
  bias_1 : Constant
  bias_2 : Constant  Value=2
  coff : Constant  Value=1.5
  r2 : Math  Operator=square
  r4 : Math  Operator=square
  r5 : Product
  sub-1 : Sum  Inputs=|+-
  sub-2 : Sum  Inputs=|+-
  times_5 : Gain  Gain=5
  z2 : Math  Operator=square
  z2/r2 : Product  Inputs=*/
  防除零 : Saturate  UpperLimit=inf  LowerLimit=Re+80e3
  J2x : Outport
  J2y : Outport  Port=2
  J2z : Outport  Port=3
  wires:
  Re2/1 -> Product/2
  z2/1 -> z2/r2/1
  x轴坐标/1 -> J2_x/1
  z2/r2/1 -> times_5/1
  sub-1/1 -> J2_y/2, J2_x/2, sub-2/1
  Product/1 -> J2_x/3, J2_y/3, J2_z/3
  coff/1 -> Product/5
  J2_z/1 -> J2z/1
  r4/1 -> r5/1
  z轴坐标/1 -> J2_z/1, z2/1
  r2/1 -> z2/r2/2, r4/1
  球心距/1 -> 防除零/1
  bias_1/1 -> sub-1/2
  [mu] -> Product/3
  times_5/1 -> sub-1/1
  sub-2/1 -> J2_z/2
  Re/1 -> Re2/1
  y轴坐标/1 -> J2_y/1
  J2/1 -> Product/4
  r5/1 -> Product/1
  bias_2/1 -> sub-2/2
  J2_y/1 -> J2y/1
  J2_x/1 -> J2x/1
  防除零/1 -> r5/2, r2/1

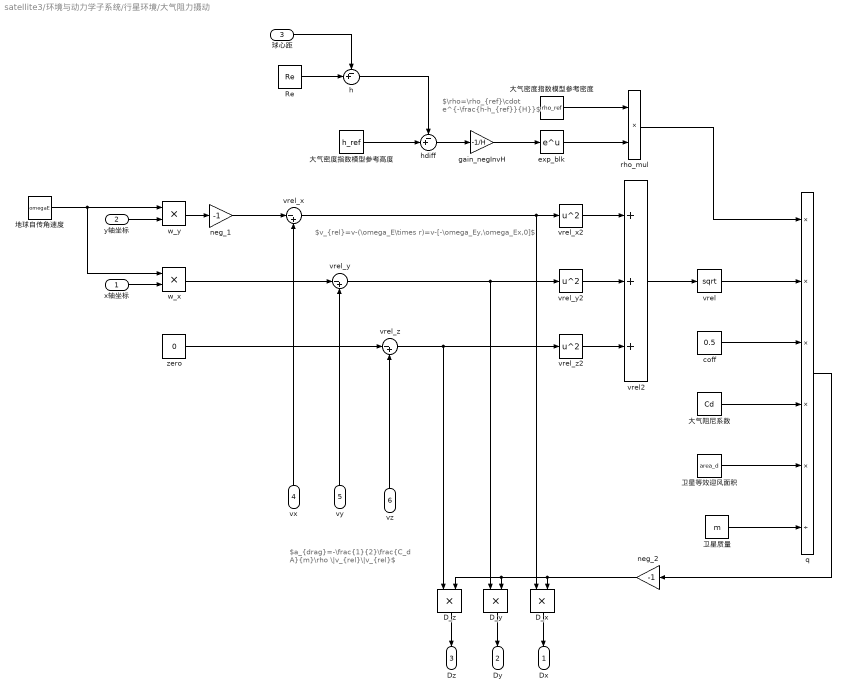
== system satellite3/环境与动力学子系统/行星环境/大气阻力摄动 ==
  note: $a_{drag}=-\frac{1}{2}\frac{C_d A}{m}\rho \|v_{rel}\|v_{rel}$
  note: $\rho=\rho_{ref}\cdot e^{-\frac{h-h_{ref}}{H}}$
  note: $v_{rel}=v-(\omega_E\times r)=v-[-\omega_Ey,\omega_Ex,0]$
  x轴坐标 : Inport
  y轴坐标 : Inport  Port=2
  球心距 : Inport  Port=3
  vx : Inport  Port=4
  vy : Inport  Port=5
  vz : Inport  Port=6
  D_x : Product
  D_y : Product
  D_z : Product
  Re : Constant  Value=Re
  coff : Constant  Value=0.5
  exp_blk : Math
  gain_negInvH : Gain  Gain=-1/H
  h : Sum  Inputs=-+|
  hdiff : Sum  Inputs=-+|
  neg_1 : Gain  Gain=-1
  neg_2 : Gain  Gain=-1
  q : Product  Inputs=*****/
  rho_mul : Product
  vrel : Sqrt
  vrel2 : Sum  Inputs=+++
  vrel_x : Sum  Inputs=|-+
  vrel_x2 : Math  Operator=square
  vrel_y : Sum  Inputs=|-+
  vrel_y2 : Math  Operator=square
  vrel_z : Sum  Inputs=|-+
  vrel_z2 : Math  Operator=square
  w_x : Product
  w_y : Product
  zero : Constant  Value=0
  卫星等效迎风面积 : Constant  Value=area_d
  卫星质量 : Constant  Value=m
  地球自传角速度 : Constant  Value=omegaE
  大气密度指数模型参考密度 : Constant  Value=rho_ref
  大气密度指数模型参考高度 : Constant  Value=h_ref
  大气阻尼系数 : Constant  Value=Cd
  Dx : Outport
  Dy : Outport  Port=2
  Dz : Outport  Port=3
  wires:
  vz/1 -> vrel_z/2
  vy/1 -> vrel_y/2
  w_y/1 -> neg_1/1
  vrel_x/1 -> D_x/1, vrel_x2/1
  q/1 -> neg_2/1
  vrel_z2/1 -> vrel2/3
  vrel_x2/1 -> vrel2/1
  大气密度指数模型参考密度/1 -> rho_mul/1
  vrel2/1 -> vrel/1
  Re/1 -> h/2
  地球自传角速度/1 -> w_x/1, w_y/1
  x轴坐标/1 -> w_x/2
  neg_1/1 -> vrel_x/1
  vrel_y/1 -> D_y/1, vrel_y2/1
  D_z/1 -> Dz/1
  vrel_y2/1 -> vrel2/2
  coff/1 -> q/3
  rho_mul/1 -> q/1
  h/1 -> hdiff/1
  w_x/1 -> vrel_y/1
  卫星质量/1 -> q/6
  卫星等效迎风面积/1 -> q/5
  gain_negInvH/1 -> exp_blk/1
  zero/1 -> vrel_z/1
  vx/1 -> vrel_x/2
  vrel_z/1 -> D_z/1, vrel_z2/1
  大气密度指数模型参考高度/1 -> hdiff/2
  hdiff/1 -> gain_negInvH/1
  vrel/1 -> q/2
  大气阻尼系数/1 -> q/4
  exp_blk/1 -> rho_mul/2
  y轴坐标/1 -> w_y/2
  球心距/1 -> h/1
  D_x/1 -> Dx/1
  D_y/1 -> Dy/1
  neg_2/1 -> D_x/2, D_y/2, D_z/2

== system satellite3/环境与动力学子系统/行星环境/太阳光压摄动 ==
  sun_flag : Inport
  hat_r_ss : Inport  Port=2
  Demux : Demux  Outputs=3
  Product : Product  Inputs=***/**
  卫星总质量 : Constant  Value=m
  受照面积 : Constant  Value=area_s
  太阳辐射压强 : Constant  Value=P0
  辐射压系数 : Constant  Value=Cr
  srp_x : Outport
  srp_y : Outport  Port=2
  srp_z : Outport  Port=3
  wires:
  hat_r_ss/1 -> Product/5
  太阳辐射压强/1 -> Product/1
  卫星总质量/1 -> Product/4
  受照面积/1 -> Product/3
  辐射压系数/1 -> Product/2
  Product/1 -> Demux/1
  Demux/3 -> srp_z/1
  Demux/2 -> srp_y/1
  Demux/1 -> srp_x/1
  sun_flag/1 -> Product/6

== system satellite3/电源子系统/太阳能板/太阳板 ==
  note: 日照期若母线电压被电池/控制抬得过高，PV 可能进入反向区（器件模型允许 I<0）
      | 真实卫星电源一般会有防反/输入级，系统级通常要求：
      | PV 对母线电流 不允许为负 （或几乎不允许）
  note: 日照期 $I_{pv}>0$ ，地影期 $I_{pv}=0$ 做成硬切换，电流是阶跃：
      | 入影瞬间： $I_{pv}$ ​ 从某值跳到 0 → $C\dot V$ 瞬间变负 → Vbus 出现尖降
      | 出影瞬间：反过来尖升
      | 因此对I_ph添加滤波
  q : Inport
  日照标志 : Inport  Port=2
  星日单位矢量 : Inport  Port=3
  母线电压 : Inport  Port=4
  Max : MinMax  Function=max  Inputs=2
  Max1 : MinMax  Function=max  Inputs=2
  Saturation : Saturate  UpperLimit=8  LowerLimit=0
  Scope1 : Scope
      settings: ActiveDisplayYMinimum=-69.050382841739946  ActiveDisplayYMaximum=15.23607432561499  DataLoggingVariableName=ScopeData41
  Scope2 : Scope
      settings: ActiveDisplayYMinimum=-2.0072254474235365  ActiveDisplayYMaximum=8.0853829043964343  DataLoggingVariableName=ScopeData42
  Scope3 : Scope  NumInputPorts=2
      settings: ActiveDisplayYMinimum=-0.13642131979695429  ActiveDisplayYMaximum=1.1760786802030458  DataLoggingVariableName=ScopeData46
  eta : Gain  Gain=eta_buck
  伏电特性 : Subsystem
  入射角余弦 : Subsystem
  入射辐照度 : Switch  Criteria=u2 ~= 0  SaturateOnIntegerOverflow=off  InputSameDT=off
  太阳翼故障 : Subsystem
  最简单光生模型 : Gain  Gain=G0
  步进MPPT : Subsystem
  太阳板输出电流 : Outport
  wires:
  最简单光生模型/1 -> 入射辐照度/1  "I_ph"
  q/1 -> 入射角余弦/1(q)
  入射角余弦/1(入射角余弦) -> Scope3/2, 最简单光生模型/1
  [zero] -> Max/2, Max1/2, 入射辐照度/3
  Max/1 -> eta/1  "I_panel"
  步进MPPT/1(太阳电池电压) -> 伏电特性/2(V)
  星日单位矢量/1 -> 入射角余弦/2(星日单位矢量)
  eta/1 -> Max1/1
  Max1/1 -> Saturation/1
  日照标志/1 -> Scope3/1, 入射辐照度/2
  入射辐照度/1 -> 伏电特性/1(lr)
  伏电特性/1(I) -> Scope1/1, 太阳翼故障/1(原值)
  Saturation/1 -> 步进MPPT/1(I_panel), Scope2/1, 太阳板输出电流/1
  母线电压/1 -> 步进MPPT/2(母线电压)
  太阳翼故障/1(故障值) -> Max/1

== system satellite3/电源子系统/太阳能板/母线故障 ==
  原值 : Inport
  Add : Sum  Inputs=2
  Sum : Sum  Inputs=|++
  偏差故障 : Subsystem
  掉线故障 : Subsystem
  故障值 : Outport
  wires:
  掉线故障/1(故障值注入) -> Add/2
  偏差故障/1(故障值注入) -> Add/1
  Add/1 -> Sum/2
  Sum/1 -> 故障值/1
  原值/1 -> Sum/1, 掉线故障/1(原值)

== system satellite3/电源子系统/蓄电池组/蓄电池组故障 ==
  原值 : Inport
  Add : Sum
  Sum : Sum  Inputs=|++
  乘性故障 : Subsystem
  偏差故障 : Subsystem
  故障值 : Outport
  wires:
  乘性故障/1(故障值注入) -> Add/2
  Sum/1 -> 故障值/1
  原值/1 -> Sum/1, 乘性故障/1(原值)
  偏差故障/1(故障值注入) -> Add/1
  Add/1 -> Sum/2

== system satellite3/姿态确定与控制系统/三轴PD控制器/四元数归一化/向量模长-q ==
  u0 : Inport
  u1 : Inport  Port=2
  u2 : Inport  Port=3
  u3 : Inport  Port=4
  Add : Sum  Inputs=4
  Sqrt : Sqrt
  Square{,1..3} (4 alike) : Math  Operator=square
  |u| : Outport
  wires:
  u0/1 -> Square/1
  u1/1 -> Square1/1
  u2/1 -> Square2/1
  Square/1 -> Add/1
  Square1/1 -> Add/2
  Square2/1 -> Add/3
  Add/1 -> Sqrt/1
  Sqrt/1 -> |u|/1
  u3/1 -> Square3/1
  Square3/1 -> Add/4

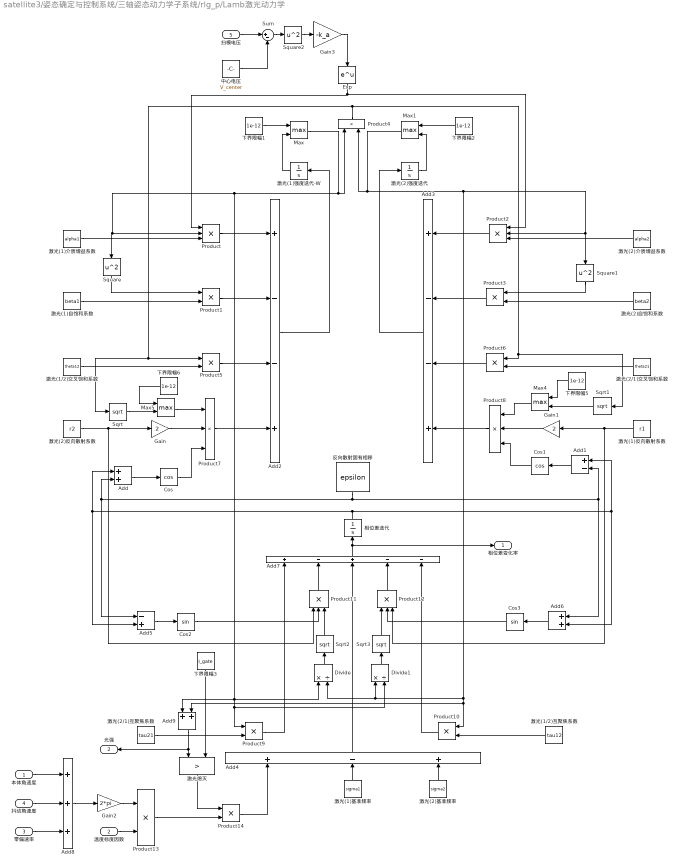
== system satellite3/姿态确定与控制系统/三轴姿态动力学子系统/rlg_p/Lamb激光动力学 ==
  本体角速度 : Inport
  温度标度因数 : Inport  Port=2
  零偏速率 : Inport  Port=3
  抖动角速度 : Inport  Port=4
  扫模电压 : Inport  Port=5
  Add : Sum
  Add1 : Sum  Inputs=+-
  Add2 : Sum  Inputs=+--+
  Add3 : Sum  Inputs=+--+
  Add4 : Sum  Inputs=+-+
  Add5 : Sum  Inputs=-+
  Add6 : Sum
  Add7 : Sum  Inputs=+-+--
  Add8 : Sum  Inputs=+++
  Add9 : Sum
  Cos : Trigonometry  Operator=cos
  Cos1 : Trigonometry  Operator=cos
  Cos2 : Trigonometry
  Cos3 : Trigonometry
  Divide : Product  Inputs=*/
  Divide1 : Product  Inputs=*/
  Exp : Math
  Gain : Gain  Gain=2
  Gain1 : Gain  Gain=2
  Gain2 : Gain  Gain=2*pi
  Gain3 : Gain  Gain=-k_a
  Max{,1,4..5} (4 alike) : MinMax  Function=max  Inputs=2
  Product{,2,7..8,11..12} (6 alike) : Product  Inputs=3
  Product{1,3..6,9..10,13..14} (9 alike) : Product
  Sqrt{,1..3} (4 alike) : Sqrt
  Square : Math  Operator=square
  Square1 : Math  Operator=square
  Square2 : Math  Operator=square
  Sum : Sum  Inputs=|+-
  下界限幅{1..2,5..6} (4 alike) : Constant  Value=1e-12
  下界限幅3 : Constant  Value=I_gate
  中心电压 : Constant  Value=V_center
  反向散射固有相移 : Constant  Value=epsilon
  激光(1)介质增益系数 : Constant  Value=alpha1
  激光(1)反向散射系数 : Constant  Value=r1
  激光(1)基准频率 : Constant  Value=sigma1
  激光(1)强度迭代-W : Integrator  InitialCondition=1
  激光(1)自饱和系数 : Constant  Value=beta1
  激光(1/2)互聚焦系数 : Constant  Value=tau12
  激光(1/2)交叉饱和系数 : Constant  Value=theta12
  激光(2)介质增益系数 : Constant  Value=alpha2
  激光(2)反向散射系数 : Constant  Value=r2
  激光(2)基准频率 : Constant  Value=sigma2
  激光(2)强度迭代 : Integrator  InitialCondition=1
  激光(2)自饱和系数 : Constant  Value=beta2
  激光(2/1)互聚焦系数 : Constant  Value=tau21
  激光(2/1)交叉饱和系数 : Constant  Value=theta21
  激光熄灭 : RelationalOperator  Operator=>  OutDataTypeStr=boolean  InputSameDT=off
  相位差迭代 : Integrator
  相位差变化率 : Outport
  光强 : Outport  Port=2
  wires:
  激光(1)介质增益系数/1 -> Product/3
  激光(1)自饱和系数/1 -> Product1/2
  Square/1 -> Product1/1
  激光(2)介质增益系数/1 -> Product2/3
  激光(2)自饱和系数/1 -> Product3/2
  Square1/1 -> Product3/1
  激光(1/2)交叉饱和系数/1 -> Product5/2
  激光(2/1)交叉饱和系数/1 -> Product6/2
  下界限幅1/1 -> Max/1
  Product4/1 -> Product6/1, Sqrt1/1, Product5/1, Sqrt/1
  激光(2)反向散射系数/1 -> Gain/1, Product11/1
  Gain/1 -> Product7/2
  Max5/1 -> Product7/1
  Cos/1 -> Product7/3
  Add/1 -> Cos/1
  反向散射固有相移/1 -> Add1/2, Add6/1, Add5/1, Add/2
  Cos1/1 -> Product8/3
  Max4/1 -> Product8/1
  Add1/1 -> Cos1/1
  Gain1/1 -> Product8/2
  激光(1)反向散射系数/1 -> Product12/3, Gain1/1
  下界限幅2/1 -> Max1/1
  Product/1 -> Add2/1
  Product1/1 -> Add2/2
  Product5/1 -> Add2/3
  Add2/1 -> 激光(1)强度迭代-W/1
  Product2/1 -> Add3/1
  Product3/1 -> Add3/2
  Product6/1 -> Add3/3
  Product8/1 -> Add3/4
  Add3/1 -> 激光(2)强度迭代/1
  激光(2/1)互聚焦系数/1 -> Product9/2
  激光(1/2)互聚焦系数/1 -> Product10/2
  Product7/1 -> Add2/4
  Add5/1 -> Cos2/1
  Max/1 -> Add9/1, Product9/1, Divide1/2, Divide/1, Product/2, Square/1, Product4/1
  Divide/1 -> Sqrt2/1
  Cos2/1 -> Product11/2
  相位差迭代/1 -> Add1/1, Add6/2, Add5/2, Add/1
  Add6/1 -> Cos3/1
  Divide1/1 -> Sqrt3/1
  Cos3/1 -> Product12/2
  激光(1)基准频率/1 -> Add4/2
  激光(2)基准频率/1 -> Add4/3
  Product14/1 -> Add4/1
  Product9/1 -> Add7/1
  Product10/1 -> Add7/5
  Product11/1 -> Add7/2
  Product12/1 -> Add7/4
  Add4/1 -> Add7/3
  Add7/1 -> 相位差变化率/1, 相位差迭代/1
  激光(1)强度迭代-W/1 -> Max/2
  激光(2)强度迭代/1 -> Max1/2
  下界限幅5/1 -> Max4/1
  Sqrt1/1 -> Max4/2
  下界限幅6/1 -> Max5/1
  Sqrt/1 -> Max5/2
  Sqrt2/1 -> Product11/3
  Sqrt3/1 -> Product12/1
  零偏速率/1 -> Add8/3
  温度标度因数/1 -> Product13/2
  本体角速度/1 -> Add8/1
  抖动角速度/1 -> Add8/2
  Add8/1 -> Gain2/1
  Gain2/1 -> Product13/1
  Max1/1 -> Product4/2, Square1/1, Product2/2, Divide/2, Divide1/1, Add9/2, Product10/1
  Add9/1 -> 光强/1, 激光熄灭/1
  Product13/1 -> Product14/2
  激光熄灭/1 -> Product14/1
  下界限幅3/1 -> 激光熄灭/2
  扫模电压/1 -> Sum/1
  中心电压/1 -> Sum/2
  Sum/1 -> Square2/1
  Gain3/1 -> Exp/1
  Exp/1 -> Product2/1, Product/1
  Square2/1 -> Gain3/1

== system satellite3/姿态确定与控制系统/三轴姿态动力学子系统/rlg_p/几何参数 ==
  Mux : Mux  Inputs=3
  激光波长-m : Constant  Value=wavelength_m
  环形腔周长-m : Constant  Value=perimeter_m
  环形腔面积-m2 : Constant  Value=area_m2
  计算集合标度因数-S0 : Fcn  Expr=4*u(1)/(u(2)*u(3))
  标度因数 : Outport
  wires:
  计算集合标度因数-S0/1 -> 标度因数/1
  Mux/1 -> 计算集合标度因数-S0/1
  环形腔面积-m2/1 -> Mux/1
  激光波长-m/1 -> Mux/2
  环形腔周长-m/1 -> Mux/3

== system satellite3/姿态确定与控制系统/三轴姿态动力学子系统/rlg_p/噪声模型 ==
  标度因数 : Inport
  相位差变化率 : Inport  Port=2
  Add : Sum
  Band-Limited White Noise : simulink/Sources/Band-Limited White Noise  Cov=[(ARW_deg_per_sqrt_h/60)^2 + white_rate_std_deg_s^2]  Ts=1  seed=[23341]
  Divide : Product  Inputs=/*
  Gain : Gain  Gain=pi/180
  r2Hz : Gain  Gain=1/(2*pi)
  测量角速度 : Outport
  wires:
  Add/1 -> 测量角速度/1
  r2Hz/1 -> Divide/2
  Gain/1 -> Add/1
  Band-Limited White Noise/1 -> Gain/1
  Divide/1 -> Add/2
  相位差变化率/1 -> r2Hz/1
  标度因数/1 -> Divide/1

== system satellite3/姿态确定与控制系统/三轴姿态动力学子系统/rlg_p/控模与扫模逻辑 ==
  光强 : Inport
  Add : Sum  Inputs=+-
  Add1 : Sum
  Gain : Gain  Gain=kP
  Gain1 : Gain  Gain=kI
  Integrator : Integrator
  Switch : Switch  Criteria=u2 > Threshold  SaturateOnIntegerOverflow=off  InputSameDT=off
  zero : Constant  Value=0  OutDataTypeStr=boolean
  光强阈值 : Constant  Value=I_triggle
  扫模信号发生器 : simulink/Sources/Repeating Sequence  rep_seq_t=[0 0.5 1]  rep_seq_y=[0 V_pzt_max V_pzt_min]
  期望光强 : Constant  Value=I_e
  状态切换 : simulink_extras/Flip Flops/S-R Flip-Flop  initial_condition=0
  触发信号 : RelationalOperator  OutDataTypeStr=boolean  RndMeth=Simplest  InputSameDT=off
  触发信号1 : RelationalOperator  Operator=<  OutDataTypeStr=boolean  RndMeth=Simplest  InputSameDT=off
  跌落阈值 : Constant  Value=I_gate
  扫模电压 : Outport
  wires:
  光强阈值/1 -> 触发信号/2
  期望光强/1 -> Add/1
  Add1/1 -> Switch/1
  状态切换/1 -> Switch/2
  扫模信号发生器/1 -> Switch/3
  触发信号/1 -> 状态切换/1
  Switch/1 -> 扫模电压/1
  Add/1 -> Gain1/1, Gain/1
  Gain/1 -> Add1/2
  Gain1/1 -> Integrator/1
  Integrator/1 -> Add1/1
  触发信号1/1 -> 状态切换/2
  光强/1 -> 触发信号1/1, Add/2, 触发信号/1
  跌落阈值/1 -> 触发信号1/2

== system satellite3/姿态确定与控制系统/三轴姿态动力学子系统/rlg_p/机械抖动 ==
  Add : Sum
  Add1 : Sum  Inputs=-+-
  Clock : Clock
  Product{,1..3,5} (5 alike) : Product
  Product6 : Product  Inputs=3
  Scope : Scope
      settings: DataLoggingVariableName=ScopeData4
  Scope1 : Scope
      settings: DataLoggingVariableName=ScopeData5
  Sin : Trigonometry
  Square : Math  Operator=square
  deg2rad : Gain  Gain=pi/180
  dither_d : ToWorkspace  VariableName=dither_d  SampleTime=-1
  dither_w : ToWorkspace  VariableName=dither_w  SampleTime=-1
  r2rad : Gain  Gain=2*pi
  倍数 : Constant  Value=2.0
  初相位 : Constant  Value=initial_phase
  抖动固有频率-Hz : Constant  Value=f_n_hz
  抖动角度迭代 : Integrator
  抖动角速度迭代 : Integrator
  抖动角速度（峰值）-deg/s : Constant  Value=v_peak_deg_s
  阻尼比 : Constant  Value=zeta
  抖动角速度 : Outport
  wires:
  r2rad/1 -> Square/1, Product6/1, Product1/2  "抖动固有角频率-rad/s"
  抖动固有频率-Hz/1 -> r2rad/1
  阻尼比/1 -> Product/2
  倍数/1 -> Product/1
  Clock/1 -> Product1/1
  Product1/1 -> Add/1
  初相位/1 -> Add/2
  Add/1 -> Sin/1
  Product3/1 -> Product2/1  "驱动力矩幅值-N·m"
  Sin/1 -> Product2/2
  Product2/1 -> Add1/2  "驱动力矩-N·m"
  deg2rad/1 -> Product3/1  "抖动角度幅值-rad"
  抖动角速度（峰值）-deg/s/1 -> deg2rad/1
  Product/1 -> Product6/2, Product3/2
  Add1/1 -> 抖动角速度迭代/1
  Product6/1 -> Add1/3
  Square/1 -> Product5/2
  抖动角度迭代/1 -> dither_d/1, Scope1/1, Product5/1
  Product5/1 -> Add1/1
  抖动角速度迭代/1 -> Scope/1, dither_w/1, Product6/3, 抖动角速度/1, 抖动角度迭代/1

== system satellite3/姿态确定与控制系统/三轴姿态动力学子系统/rlg_p/热模型 ==
  环境温度-°C : Inport
  几何标度因数 : Inport  Port=2
  Add : Sum
  Add1 : Sum  Inputs=+++
  Add2 : Sum
  Product : Product
  Sum : Sum  Inputs=|-+
  deg2rad(s) : Gain  Gain=pi/(180*3600)
  平方 : Math  Operator=square
  标定/初始温度 : Constant  Value=25
  标度因数倍数（参考温度） : Constant
  比较 : Sum  Inputs=-+|
  温度标度因数系数（1阶） : Gain  Gain=k_sf1_ppm
  温度标度因数系数（2阶） : Gain  Gain=k_sf2_ppm
  温度迭代 : Integrator  InitialConditionSource=external  InitialCondition=25.0
  温度零偏系数（1阶） : Gain  Gain=k_bias1_deg_h_per_C
  温度零偏系数（2阶） : Gain  Gain=k_bias2_deg_h_per_C
  热时间常数 : Gain  Gain=1/tau_th_s
  百万分之一每摄氏度 : Gain  Gain=1e-6
  零偏（参考温度） : Constant  Value=bias0_deg_h
  陀螺温度-°C : Outport
  温度标度因数 : Outport  Port=2
  温度零偏 : Outport  Port=3
  wires:
  热时间常数/1 -> 温度迭代/1
  温度迭代/1 -> 陀螺温度-°C/1, Sum/2, 比较/1
  环境温度-°C/1 -> 比较/2
  比较/1 -> 热时间常数/1
  温度标度因数系数（1阶）/1 -> Add/1
  温度标度因数系数（2阶）/1 -> Add/2
  标定/初始温度/1 -> Sum/1, 温度迭代/2
  Add/1 -> 百万分之一每摄氏度/1
  Product/1 -> 温度标度因数/1
  平方/1 -> 温度标度因数系数（2阶）/1, 温度零偏系数（2阶）/1
  deg2rad(s)/1 -> 温度零偏/1
  几何标度因数/1 -> Product/1
  Add1/1 -> deg2rad(s)/1
  Sum/1 -> 平方/1, 温度标度因数系数（1阶）/1, 温度零偏系数（1阶）/1
  温度零偏系数（2阶）/1 -> Add1/3
  温度零偏系数（1阶）/1 -> Add1/2
  零偏（参考温度）/1 -> Add1/1
  百万分之一每摄氏度/1 -> Add2/2
  标度因数倍数（参考温度）/1 -> Add2/1
  Add2/1 -> Product/2

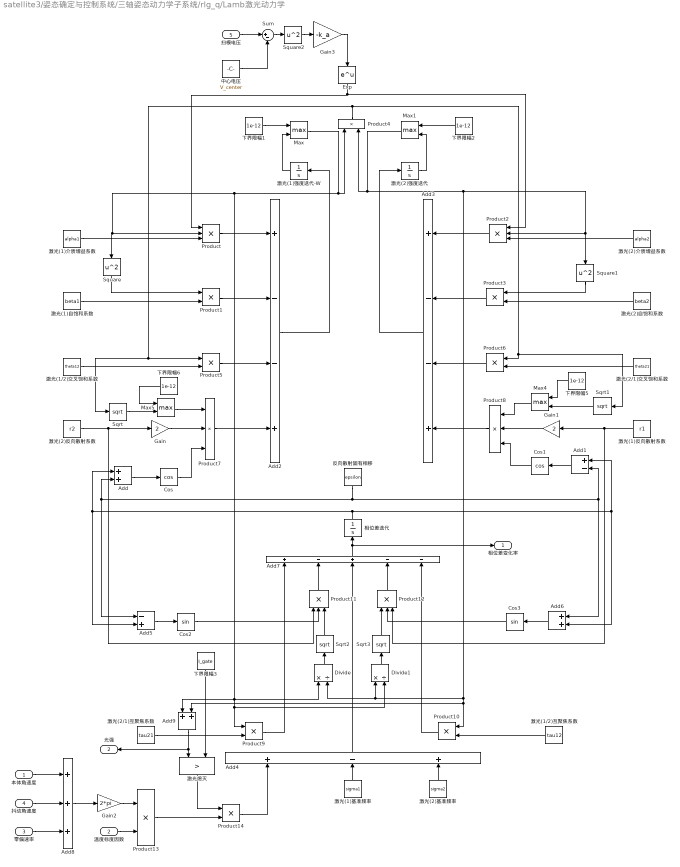
== system satellite3/姿态确定与控制系统/三轴姿态动力学子系统/rlg_q/Lamb激光动力学 ==
  本体角速度 : Inport
  温度标度因数 : Inport  Port=2
  零偏速率 : Inport  Port=3
  抖动角速度 : Inport  Port=4
  扫模电压 : Inport  Port=5
  Add : Sum
  Add1 : Sum  Inputs=+-
  Add2 : Sum  Inputs=+--+
  Add3 : Sum  Inputs=+--+
  Add4 : Sum  Inputs=+-+
  Add5 : Sum  Inputs=-+
  Add6 : Sum
  Add7 : Sum  Inputs=+-+--
  Add8 : Sum  Inputs=+++
  Add9 : Sum
  Cos : Trigonometry  Operator=cos
  Cos1 : Trigonometry  Operator=cos
  Cos2 : Trigonometry
  Cos3 : Trigonometry
  Divide : Product  Inputs=*/
  Divide1 : Product  Inputs=*/
  Exp : Math
  Gain : Gain  Gain=2
  Gain1 : Gain  Gain=2
  Gain2 : Gain  Gain=2*pi
  Gain3 : Gain  Gain=-k_a
  Max{,1,4..5} (4 alike) : MinMax  Function=max  Inputs=2
  Product{,2,7..8,11..12} (6 alike) : Product  Inputs=3
  Product{1,3..6,9..10,13..14} (9 alike) : Product
  Sqrt{,1..3} (4 alike) : Sqrt
  Square : Math  Operator=square
  Square1 : Math  Operator=square
  Square2 : Math  Operator=square
  Sum : Sum  Inputs=|+-
  下界限幅{1..2,5..6} (4 alike) : Constant  Value=1e-12
  下界限幅3 : Constant  Value=I_gate
  中心电压 : Constant  Value=V_center
  反向散射固有相移 : Constant  Value=epsilon
  激光(1)介质增益系数 : Constant  Value=alpha1
  激光(1)反向散射系数 : Constant  Value=r1
  激光(1)基准频率 : Constant  Value=sigma1
  激光(1)强度迭代-W : Integrator  InitialCondition=1
  激光(1)自饱和系数 : Constant  Value=beta1
  激光(1/2)互聚焦系数 : Constant  Value=tau12
  激光(1/2)交叉饱和系数 : Constant  Value=theta12
  激光(2)介质增益系数 : Constant  Value=alpha2
  激光(2)反向散射系数 : Constant  Value=r2
  激光(2)基准频率 : Constant  Value=sigma2
  激光(2)强度迭代 : Integrator  InitialCondition=1
  激光(2)自饱和系数 : Constant  Value=beta2
  激光(2/1)互聚焦系数 : Constant  Value=tau21
  激光(2/1)交叉饱和系数 : Constant  Value=theta21
  激光熄灭 : RelationalOperator  Operator=>  OutDataTypeStr=boolean  InputSameDT=off
  相位差迭代 : Integrator
  相位差变化率 : Outport
  光强 : Outport  Port=2
  wires:
  Square2/1 -> Gain3/1
  Exp/1 -> Product/1, Product2/1
  Gain3/1 -> Exp/1
  Sum/1 -> Square2/1
  中心电压/1 -> Sum/2
  扫模电压/1 -> Sum/1
  下界限幅3/1 -> 激光熄灭/2
  激光熄灭/1 -> Product14/1
  Product13/1 -> Product14/2
  Add9/1 -> 激光熄灭/1, 光强/1
  Max1/1 -> Product10/1, Add9/2, Divide1/1, Divide/2, Product2/2, Square1/1, Product4/2
  Gain2/1 -> Product13/1
  Add8/1 -> Gain2/1
  抖动角速度/1 -> Add8/2
  本体角速度/1 -> Add8/1
  温度标度因数/1 -> Product13/2
  零偏速率/1 -> Add8/3
  Sqrt3/1 -> Product12/1
  Sqrt2/1 -> Product11/3
  Sqrt/1 -> Max5/2
  下界限幅6/1 -> Max5/1
  Sqrt1/1 -> Max4/2
  下界限幅5/1 -> Max4/1
  激光(2)强度迭代/1 -> Max1/2
  激光(1)强度迭代-W/1 -> Max/2
  Add7/1 -> 相位差迭代/1, 相位差变化率/1
  Add4/1 -> Add7/3
  Product12/1 -> Add7/4
  Product11/1 -> Add7/2
  Product10/1 -> Add7/5
  Product9/1 -> Add7/1
  Product14/1 -> Add4/1
  激光(2)基准频率/1 -> Add4/3
  激光(1)基准频率/1 -> Add4/2
  Cos3/1 -> Product12/2
  Divide1/1 -> Sqrt3/1
  Add6/1 -> Cos3/1
  相位差迭代/1 -> Add/1, Add5/2, Add6/2, Add1/1
  Cos2/1 -> Product11/2
  Divide/1 -> Sqrt2/1
  Max/1 -> Product4/1, Square/1, Product/2, Divide/1, Divide1/2, Product9/1, Add9/1
  Add5/1 -> Cos2/1
  Product7/1 -> Add2/4
  激光(1/2)互聚焦系数/1 -> Product10/2
  激光(2/1)互聚焦系数/1 -> Product9/2
  Add3/1 -> 激光(2)强度迭代/1
  Product8/1 -> Add3/4
  Product6/1 -> Add3/3
  Product3/1 -> Add3/2
  Product2/1 -> Add3/1
  Add2/1 -> 激光(1)强度迭代-W/1
  Product5/1 -> Add2/3
  Product1/1 -> Add2/2
  Product/1 -> Add2/1
  下界限幅2/1 -> Max1/1
  激光(1)反向散射系数/1 -> Gain1/1, Product12/3
  Gain1/1 -> Product8/2
  Add1/1 -> Cos1/1
  Max4/1 -> Product8/1
  Cos1/1 -> Product8/3
  反向散射固有相移/1 -> Add/2, Add5/1, Add6/1, Add1/2
  Add/1 -> Cos/1
  Cos/1 -> Product7/3
  Max5/1 -> Product7/1
  Gain/1 -> Product7/2
  激光(2)反向散射系数/1 -> Product11/1, Gain/1
  Product4/1 -> Sqrt/1, Product5/1, Sqrt1/1, Product6/1
  下界限幅1/1 -> Max/1
  激光(2/1)交叉饱和系数/1 -> Product6/2
  激光(1/2)交叉饱和系数/1 -> Product5/2
  Square1/1 -> Product3/1
  激光(2)自饱和系数/1 -> Product3/2
  激光(2)介质增益系数/1 -> Product2/3
  Square/1 -> Product1/1
  激光(1)自饱和系数/1 -> Product1/2
  激光(1)介质增益系数/1 -> Product/3

== system satellite3/姿态确定与控制系统/三轴姿态动力学子系统/rlg_q/几何参数 ==
  Mux : Mux  Inputs=3
  激光波长-m : Constant  Value=wavelength_m
  环形腔周长-m : Constant  Value=perimeter_m
  环形腔面积-m2 : Constant  Value=area_m2
  计算集合标度因数-S0 : Fcn  Expr=4*u(1)/(u(2)*u(3))
  标度因数 : Outport
  wires:
  环形腔周长-m/1 -> Mux/3
  激光波长-m/1 -> Mux/2
  环形腔面积-m2/1 -> Mux/1
  Mux/1 -> 计算集合标度因数-S0/1
  计算集合标度因数-S0/1 -> 标度因数/1

== system satellite3/姿态确定与控制系统/三轴姿态动力学子系统/rlg_q/噪声模型 ==
  标度因数 : Inport
  相位差变化率 : Inport  Port=2
  Add : Sum
  Band-Limited White Noise : simulink/Sources/Band-Limited White Noise  Cov=[(ARW_deg_per_sqrt_h/60)^2 + white_rate_std_deg_s^2]  Ts=1  seed=[23341]
  Divide : Product  Inputs=/*
  Gain : Gain  Gain=pi/180
  r2Hz : Gain  Gain=1/(2*pi)
  测量角速度 : Outport
  wires:
  标度因数/1 -> Divide/1
  相位差变化率/1 -> r2Hz/1
  Divide/1 -> Add/2
  Band-Limited White Noise/1 -> Gain/1
  Gain/1 -> Add/1
  r2Hz/1 -> Divide/2
  Add/1 -> 测量角速度/1
